simulink model "phasedArrayBeamformer_test"  (R2019b)
settings: Solver=VariableStepAuto  StartTime=0.0  StopTime=5  RelTol=1e-3
model workspace: external: MAT-File C:\Users\jones\Documents\Repos\Infrasonic-Wave-Detection\simulink_bench.mat (data not in the file)
values from neighbouring files (symbols this model uses):
  f = p2(3)    [init_function.m]
libraries: simulink x4, hdlsllib x4
settings Model: Creator=khristian  LastModifiedBy=jones
settings DataIOCC: ReturnWorkspaceOutputs=off
settings OptimizationCC: BlockReduction=off  ConditionallyExecuteInputs=off  DefaultParameterBehavior=Inlined
settings DebuggingCC: AlgebraicLoopMsg=error  ArithmeticOperatorsInVariantConditions=warning
settings HardwareCC: ProdBitPerPointer=32  ProdBitPerSizeT=32  ProdBitPerPtrDiffT=32  ProdLargestAtomicFloat=None  ProdIntDivRoundTo=Undefined  ProdEndianess=Unspecified  ProdWordSize=32  ProdHWDeviceType=ASIC/FPGA->ASIC/FPGA  TargetBitPerPointer=64  TargetBitPerSizeT=64  TargetBitPerPtrDiffT=64  TargetLongLongMode=on  TargetIntDivRoundTo=Zero  TargetEndianess=LittleEndian  TargetWordSize=64  TargetHWDeviceType=Custom Processor->MATLAB Host Computer  ProdEqTarget=off
settings SFSimCC: CustomCodeUndefinedFunction=UseInterfaceOnly

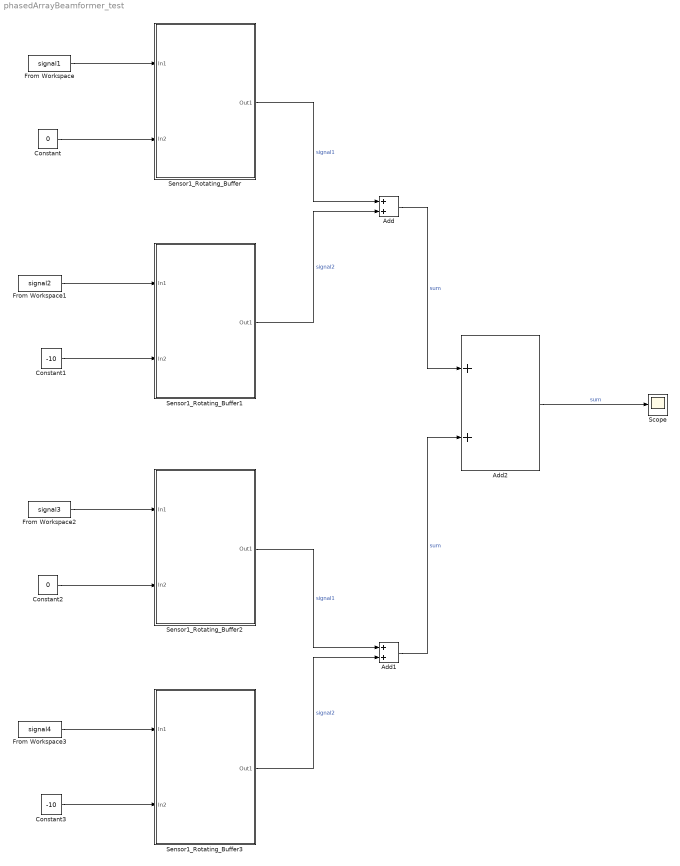
== system phasedArrayBeamformer_test ==
  Add : Sum
  Add1 : Sum
  Add2 : Sum
  Constant : Constant  Value=0
  Constant1 : Constant  Value=-10  SampleTime=-1
  Constant2 : Constant  Value=0
  Constant3 : Constant  Value=-10  SampleTime=-1
  From Workspace : FromWorkspace  VariableName=signal1  OutDataTypeStr=double
  From Workspace1 : FromWorkspace  VariableName=signal2  SampleTime=1e-3
  From Workspace2 : FromWorkspace  VariableName=signal3  OutDataTypeStr=double
  From Workspace3 : FromWorkspace  VariableName=signal4  SampleTime=1e-3
  Scope : Scope
  Sensor1_Rotating_Buffer : Subsystem
  Sensor1_Rotating_Buffer1 : Subsystem
  Sensor1_Rotating_Buffer2 : Subsystem
  Sensor1_Rotating_Buffer3 : Subsystem
  wires:
  From Workspace/1 -> Sensor1_Rotating_Buffer/1(In1)
  Constant/1 -> Sensor1_Rotating_Buffer/2(In2)
  From Workspace1/1 -> Sensor1_Rotating_Buffer1/1(In1)
  Constant1/1 -> Sensor1_Rotating_Buffer1/2(In2)
  Sensor1_Rotating_Buffer1/1(Out1) -> Add/2  "signal2"
  Sensor1_Rotating_Buffer/1(Out1) -> Add/1  "signal1"
  Add/1 -> Add2/1  "sum"
  Sensor1_Rotating_Buffer2/1(Out1) -> Add1/1  "signal1"
  Sensor1_Rotating_Buffer3/1(Out1) -> Add1/2  "signal2"
  Constant3/1 -> Sensor1_Rotating_Buffer3/2(In2)
  Add1/1 -> Add2/2  "sum"
  Constant2/1 -> Sensor1_Rotating_Buffer2/2(In2)
  From Workspace2/1 -> Sensor1_Rotating_Buffer2/1(In1)
  From Workspace3/1 -> Sensor1_Rotating_Buffer3/1(In1)
  Add2/1 -> Scope/1  "sum"

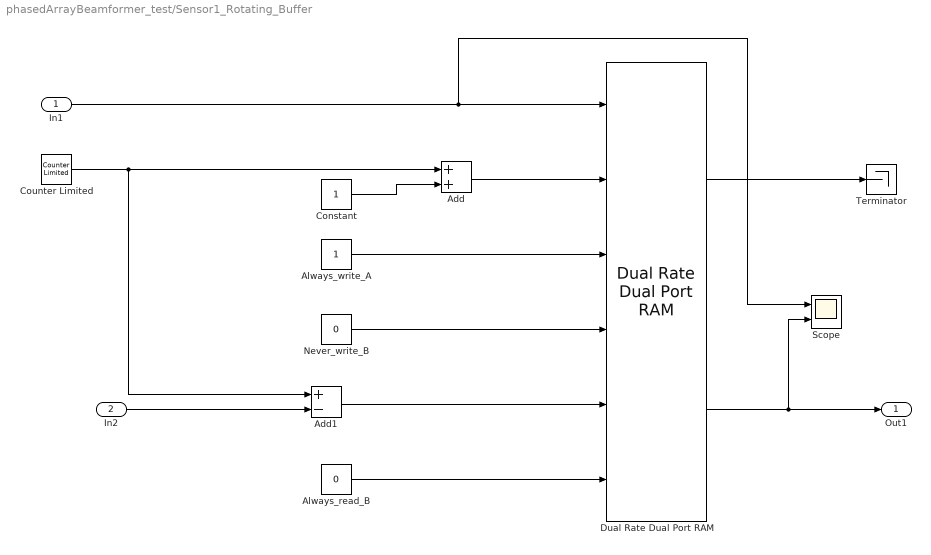
== system phasedArrayBeamformer_test/Sensor1_Rotating_Buffer ==
  In1 : Inport  OutDataTypeStr=double
  In2 : Inport  Port=2
  Add : Sum  AccumDataTypeStr=uint8  InputSameDT=on
  Add1 : Sum  Inputs=+-  AccumDataTypeStr=uint8
  Always_read_B : Constant  Value=0  OutDataTypeStr=boolean  SampleTime=-1
  Always_write_A : Constant  OutDataTypeStr=boolean  SampleTime=-1
  Constant : Constant  SampleTime=-1
  Counter Limited : simulink/Sources/Counter Limited  uplimit=255  tsamp=1/f
  Dual Rate Dual Port RAM : hdlsllib/HDL RAMs/Dual Rate Dual Port RAM  ram_size=16
      settings: SourceProductName=Simulink  SourceProductBaseCode=SL
  Never_write_B : Constant  Value=0  OutDataTypeStr=double
  Scope : Scope  NumInputPorts=2
  Terminator : Terminator
  Out1 : Outport  VectorParamsAs1DForOutWhenUnconnected=off
  wires:
  In1/1 -> Scope/1, Dual Rate Dual Port RAM/1
  Dual Rate Dual Port RAM/1 -> Terminator/1
  Always_write_A/1 -> Dual Rate Dual Port RAM/3
  Never_write_B/1 -> Dual Rate Dual Port RAM/4
  Counter Limited/1 -> Add1/1, Add/1
  Always_read_B/1 -> Dual Rate Dual Port RAM/6
  Dual Rate Dual Port RAM/2 -> Scope/2, Out1/1
  Add/1 -> Dual Rate Dual Port RAM/2
  Constant/1 -> Add/2
  Add1/1 -> Dual Rate Dual Port RAM/5
  In2/1 -> Add1/2

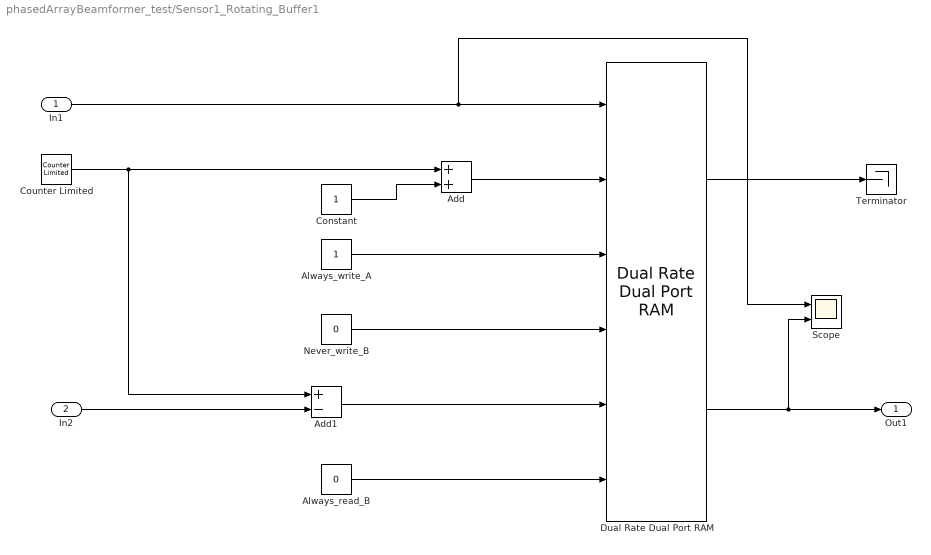
== system phasedArrayBeamformer_test/Sensor1_Rotating_Buffer1 ==
  In1 : Inport
  In2 : Inport  Port=2
  Add : Sum  AccumDataTypeStr=uint8
  Add1 : Sum  Inputs=+-  AccumDataTypeStr=uint8
  Always_read_B : Constant  Value=0  OutDataTypeStr=boolean  SampleTime=-1
  Always_write_A : Constant  OutDataTypeStr=boolean  SampleTime=-1
  Constant : Constant  SampleTime=-1
  Counter Limited : simulink/Sources/Counter Limited  uplimit=255  tsamp=1e-3
  Dual Rate Dual Port RAM : hdlsllib/HDL RAMs/Dual Rate Dual Port RAM  ram_size=8
      settings: SourceProductName=Simulink  SourceProductBaseCode=SL
  Never_write_B : Constant  Value=0  OutDataTypeStr=double
  Scope : Scope  NumInputPorts=2
  Terminator : Terminator
  Out1 : Outport  VectorParamsAs1DForOutWhenUnconnected=off
  wires:
  In1/1 -> Scope/1, Dual Rate Dual Port RAM/1
  Dual Rate Dual Port RAM/1 -> Terminator/1
  Always_write_A/1 -> Dual Rate Dual Port RAM/3
  Never_write_B/1 -> Dual Rate Dual Port RAM/4
  Counter Limited/1 -> Add1/1, Add/1
  Always_read_B/1 -> Dual Rate Dual Port RAM/6
  Dual Rate Dual Port RAM/2 -> Scope/2, Out1/1
  Add/1 -> Dual Rate Dual Port RAM/2
  Constant/1 -> Add/2
  Add1/1 -> Dual Rate Dual Port RAM/5
  In2/1 -> Add1/2

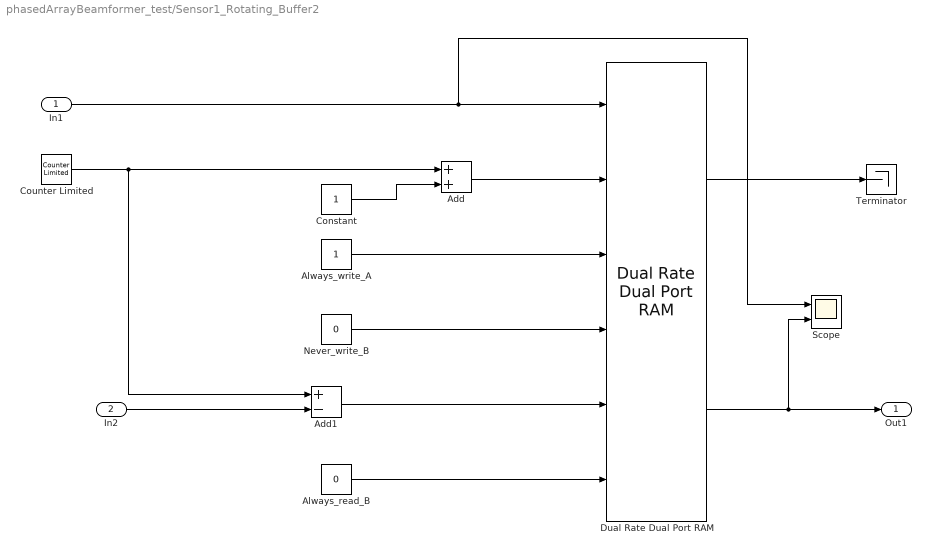
== system phasedArrayBeamformer_test/Sensor1_Rotating_Buffer2 ==
  In1 : Inport  OutDataTypeStr=double
  In2 : Inport  Port=2
  Add : Sum  AccumDataTypeStr=uint8  InputSameDT=on
  Add1 : Sum  Inputs=+-  AccumDataTypeStr=uint8
  Always_read_B : Constant  Value=0  OutDataTypeStr=boolean  SampleTime=-1
  Always_write_A : Constant  OutDataTypeStr=boolean  SampleTime=-1
  Constant : Constant  SampleTime=-1
  Counter Limited : simulink/Sources/Counter Limited  uplimit=255  tsamp=1e-3
  Dual Rate Dual Port RAM : hdlsllib/HDL RAMs/Dual Rate Dual Port RAM  ram_size=16
      settings: SourceProductName=Simulink  SourceProductBaseCode=SL
  Never_write_B : Constant  Value=0  OutDataTypeStr=double
  Scope : Scope  NumInputPorts=2
  Terminator : Terminator
  Out1 : Outport  VectorParamsAs1DForOutWhenUnconnected=off
  wires:
  In1/1 -> Scope/1, Dual Rate Dual Port RAM/1
  Dual Rate Dual Port RAM/1 -> Terminator/1
  Always_write_A/1 -> Dual Rate Dual Port RAM/3
  Never_write_B/1 -> Dual Rate Dual Port RAM/4
  Counter Limited/1 -> Add1/1, Add/1
  Always_read_B/1 -> Dual Rate Dual Port RAM/6
  Dual Rate Dual Port RAM/2 -> Scope/2, Out1/1
  Add/1 -> Dual Rate Dual Port RAM/2
  Constant/1 -> Add/2
  Add1/1 -> Dual Rate Dual Port RAM/5
  In2/1 -> Add1/2

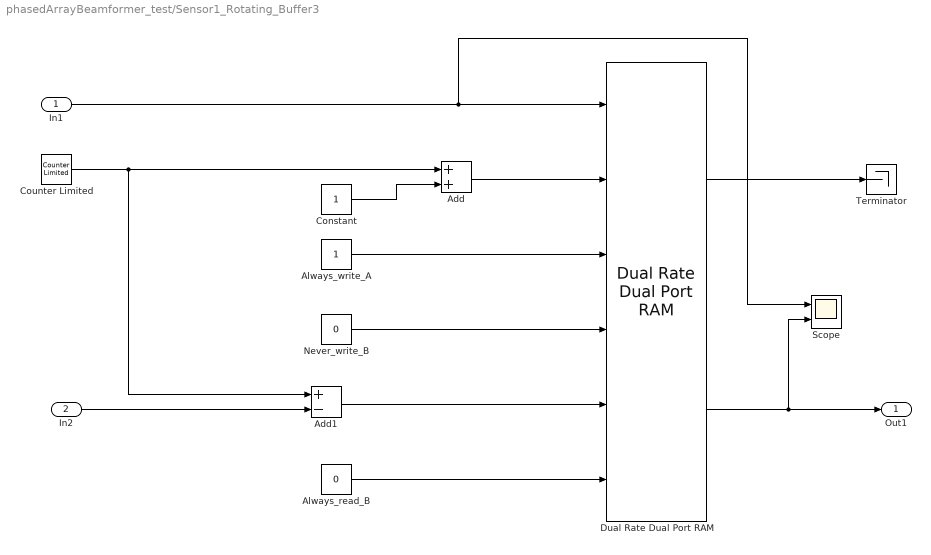
== system phasedArrayBeamformer_test/Sensor1_Rotating_Buffer3 ==
  In1 : Inport
  In2 : Inport  Port=2
  Add : Sum  AccumDataTypeStr=uint8
  Add1 : Sum  Inputs=+-  AccumDataTypeStr=uint8
  Always_read_B : Constant  Value=0  OutDataTypeStr=boolean  SampleTime=-1
  Always_write_A : Constant  OutDataTypeStr=boolean  SampleTime=-1
  Constant : Constant  SampleTime=-1
  Counter Limited : simulink/Sources/Counter Limited  uplimit=255  tsamp=1e-3
  Dual Rate Dual Port RAM : hdlsllib/HDL RAMs/Dual Rate Dual Port RAM  ram_size=8
      settings: SourceProductName=Simulink  SourceProductBaseCode=SL
  Never_write_B : Constant  Value=0  OutDataTypeStr=double
  Scope : Scope  NumInputPorts=2
  Terminator : Terminator
  Out1 : Outport  VectorParamsAs1DForOutWhenUnconnected=off
  wires:
  In1/1 -> Scope/1, Dual Rate Dual Port RAM/1
  Dual Rate Dual Port RAM/1 -> Terminator/1
  Always_write_A/1 -> Dual Rate Dual Port RAM/3
  Never_write_B/1 -> Dual Rate Dual Port RAM/4
  Counter Limited/1 -> Add1/1, Add/1
  Always_read_B/1 -> Dual Rate Dual Port RAM/6
  Dual Rate Dual Port RAM/2 -> Scope/2, Out1/1
  Add/1 -> Dual Rate Dual Port RAM/2
  Constant/1 -> Add/2
  Add1/1 -> Dual Rate Dual Port RAM/5
  In2/1 -> Add1/2
